simulink model "Lamp"  (R2018b)
settings: Solver=FixedStepDiscrete  StartTime=0.0  StopTime=30  RelTol=1e-3
settings Model: Creator=Mostafa  LastModifiedBy=Mostafa
settings ConfigSet: Description=Mostafa Hany Imam
settings OptimizationCC: DefaultParameterBehavior=Inlined  EnhancedBackFolding=on  PassReuseOutputArgsAs=Individual arguments  OptimizeBlockOrder=speed  DifferentSizesBufferReuse=on  OptimizationCustomize=off
settings DebuggingCC: UnderspecifiedInitializationDetection=Classic  MergeDetectMultiDrivingBlocksExec=none  ParameterTunabilityLossMsg=error
settings ModelReferenceCC: PropagateSignalLabelsOutOfModel=off
settings SFSimCC: MATLABDynamicMemAlloc=off
settings RTWCC: SystemTargetFile=ert.tlc  GenCodeOnly=on  TemplateMakefile=ert_default_tmf  GenerateReport=on  IncludeHyperlinkInReport=on  LaunchReport=on  GenerateTraceInfo=on  GenerateTraceReport=on  GenerateTraceReportSl=on  GenerateTraceReportSf=on  GenerateTraceReportEml=on
settings CodeAppCC: ForceParamTrailComments=on  IgnoreCustomStorageClasses=off  OperatorAnnotations=on  SimulinkDataObjDesc=on  SFDataObjDesc=on  InsertBlockDesc=on
settings ERTTargetCC: TargetLangStandard=C99 (ISO)  GenerateSampleERTMain=on  InlinedParameterPlacement=NonHierarchical  ERTCustomFileTemplate=example_file_process.tlc

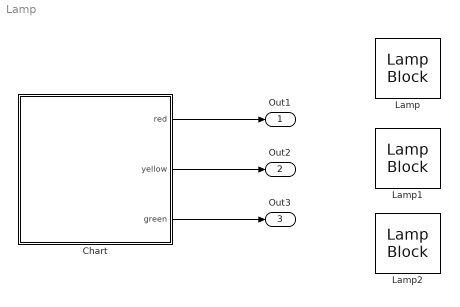
== system Lamp ==
  Chart : Stateflow chart  TreatAsAtomicUnit=on
  Lamp : LampBlock  WebBlockId=9
  Lamp1 : LampBlock  WebBlockId=10
  Lamp2 : LampBlock  WebBlockId=11
  Out1 : Outport
  Out2 : Outport  Port=2
  Out3 : Outport  Port=3
  wires:
  Chart/1(red) -> Out1/1
  Chart/2(yellow) -> Out2/1
  Chart/3(green) -> Out3/1

== stateflow chart Lamp/Chart ==
  state Yellow
    en:
    du:
    green = uint8(0);
    red = uint8(0);
    yellow =uint8(1);
    ex:
  state Green
    en:
    du:
    green =uint8(1);
    yellow = uint8(0);
    red = uint8(0);
    ex:
  state Red
    en:
    du:
    red = uint8(1);
    green = uint8(0);
    yellow = uint8(0);
    ex:
  Yellow -> Green : [after(2000,msec)]{green = uint8(0);
      | yellow = uint8(1);
      | red = uint8(0);}
  (default) -> Green
  Green -> Red : [after(5000,msec)]{green = uint8(1);
      | yellow = uint8(0);
      | red = uint8(0);
      | }
  Red -> Yellow : [after(5000,msec)]{green = uint8(0);
      | yellow = uint8(0);
      | red = uint8(1);}
  data: red output uint8; yellow output uint8; green output uint8
